simulink model "LQR_Real"  (R2022b)
settings: Solver=VariableStepAuto  StartTime=0.0  StopTime=10  RelTol=1e-3
values from neighbouring files (symbols this model uses):
  beam =     [parameters.mat]
  degs2rpm = 0.166666666667    [parameters.mat]
  Den_tm_wm = [9.422e-10 5.0182e-09 6.49379142857e-06 1.60164591837e-05]    [parameters.mat]
  der =     [parameters.mat]
  drv =     [parameters.mat]
  estimated =     [parameters.mat]
  gbox =     [parameters.mat]
  joint =     [parameters.mat]
  mot =     [parameters.mat]
  Num_tm_wm = [0.0014 0.0034 0.83]    [parameters.mat]
  rads2rpm = 9.54929658551    [parameters.mat]
  rpm2rads = 0.10471975512    [parameters.mat]
  sens =     [parameters.mat]
  Ts = 0.001    [parameters.mat]
undefined symbols (not defined in the file or in its folder): simul, ss_lqr
settings Model: Creator=emanuelevitetta  LastModifiedBy=david

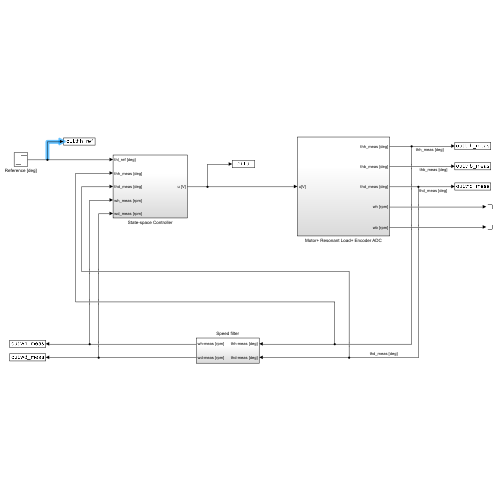
[thumbnail: Simulink's stored preview of the top-level diagram]
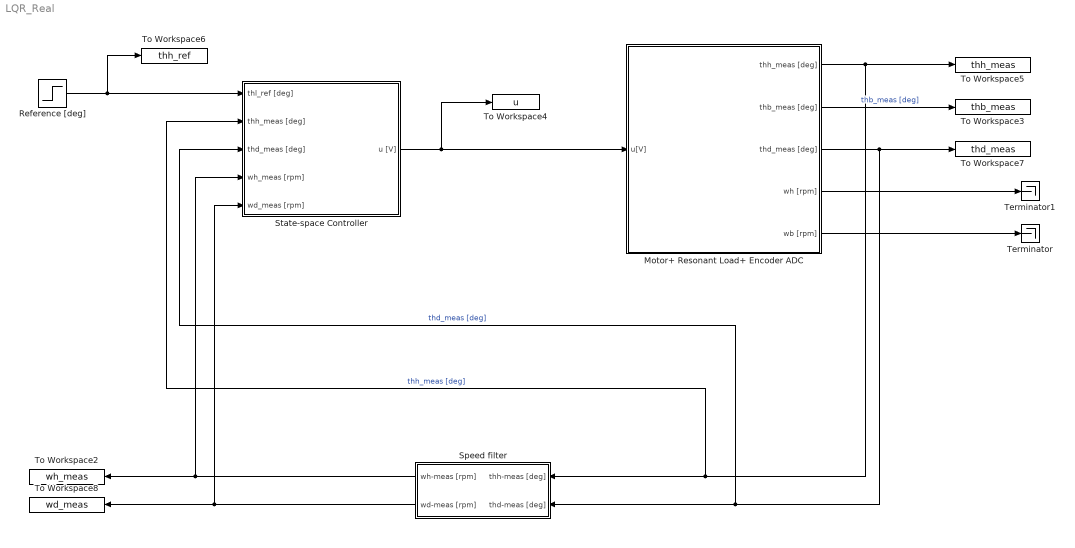
== system LQR_Real ==
  Motor+ Resonant Load+ Encoder ADC : Subsystem
  Reference [deg] : Step  After=simul.stepdeg  SampleTime=Ts
  Speed filter : Subsystem
  State-space Controller : Subsystem
  Terminator : Terminator
  Terminator1 : Terminator
  To Workspace2 : ToWorkspace  VariableName=wh_meas  SaveFormat=Structure With Time  SampleTime=Ts
  To Workspace3 : ToWorkspace  VariableName=thb_meas  SaveFormat=Structure With Time  SampleTime=Ts
  To Workspace4 : ToWorkspace  VariableName=u  SaveFormat=Structure With Time  SampleTime=Ts
  To Workspace5 : ToWorkspace  VariableName=thh_meas  SaveFormat=Structure With Time  SampleTime=Ts
  To Workspace6 : ToWorkspace  VariableName=thh_ref  SaveFormat=Structure With Time  SampleTime=-1
  To Workspace7 : ToWorkspace  VariableName=thd_meas  SaveFormat=Structure With Time  SampleTime=Ts
  To Workspace8 : ToWorkspace  VariableName=wd_meas  SaveFormat=Structure With Time  SampleTime=Ts
  wires:
  Motor+ Resonant Load+ Encoder ADC/1(thh_meas [deg]) -> State-space Controller/2(thh_meas [deg]), Speed filter/1(thh-meas [deg]), To Workspace5/1  "thh_meas [deg]"
  Motor+ Resonant Load+ Encoder ADC/2(thb_meas [deg]) -> To Workspace3/1  "thb_meas [deg]"
  State-space Controller/1(u [V]) -> Motor+ Resonant Load+ Encoder ADC/1(u[V]), To Workspace4/1
  Reference [deg]/1 -> To Workspace6/1, State-space Controller/1(thl_ref [deg])
  Motor+ Resonant Load+ Encoder ADC/5(wb [rpm]) -> Terminator/1
  Motor+ Resonant Load+ Encoder ADC/4(wh [rpm]) -> Terminator1/1
  Motor+ Resonant Load+ Encoder ADC/3(thd_meas [deg]) -> To Workspace7/1, Speed filter/2(thd-meas [deg]), State-space Controller/3(thd_meas [deg])  "thd_meas [deg]"
  Speed filter/2(wd-meas [rpm]) -> State-space Controller/5(wd_meas [rpm]), To Workspace8/1
  Speed filter/1(wh-meas [rpm]) -> State-space Controller/4(wh_meas [rpm]), To Workspace2/1

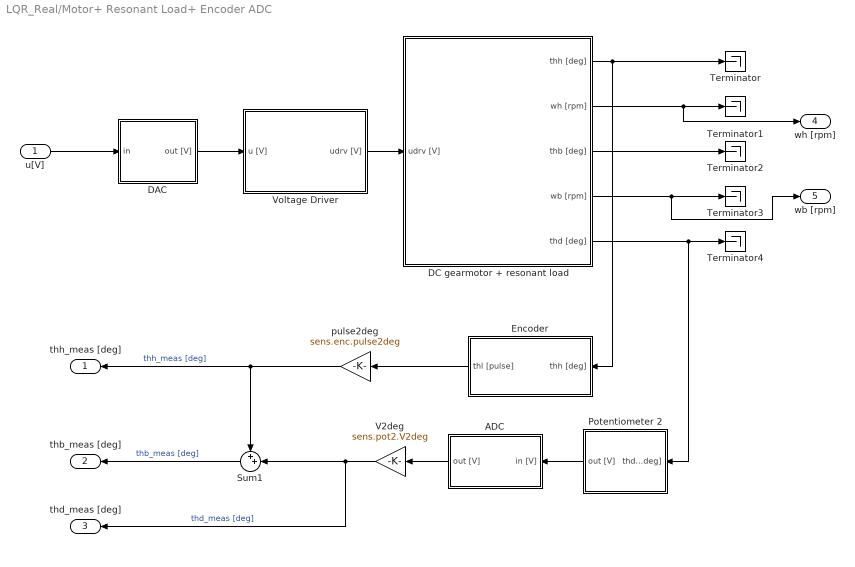
== system LQR_Real/Motor+ Resonant Load+ Encoder ADC ==
  u[V] : Inport
  ADC : Subsystem
  DAC : Subsystem
  DC gearmotor + resonant load : Subsystem
  Encoder : Subsystem
  Potentiometer 2 : Subsystem
  Sum1 : Sum  Inputs=++|
  Terminator{,1..4} (5 alike) : Terminator
  V2deg : Gain  Gain=sens.pot2.V2deg
  Voltage Driver : Subsystem
  pulse2deg : Gain  Gain=sens.enc.pulse2deg
  thh_meas [deg] : Outport
  thb_meas [deg] : Outport  Port=2
  thd_meas [deg] : Outport  Port=3
  wh [rpm] : Outport  Port=4
  wb [rpm] : Outport  Port=5
  wires:
  DC gearmotor + resonant load/2(wh [rpm]) -> wh [rpm]/1, Terminator1/1
  u[V]/1 -> DAC/1(in)
  DC gearmotor + resonant load/1(thh [deg]) -> Terminator/1, Encoder/1(thh [deg])
  DC gearmotor + resonant load/3(thb [deg]) -> Terminator2/1
  DC gearmotor + resonant load/4(wb [rpm]) -> wb [rpm]/1, Terminator3/1
  DC gearmotor + resonant load/5(thd [deg]) -> Terminator4/1, Potentiometer 2/1(thd [deg])
  DAC/1(out [V]) -> Voltage Driver/1(u [V])
  Voltage Driver/1(udrv [V]) -> DC gearmotor + resonant load/1(udrv [V])
  pulse2deg/1 -> thh_meas [deg]/1, Sum1/1  "thh_meas [deg]"
  V2deg/1 -> thd_meas [deg]/1, Sum1/2  "thd_meas [deg]"
  Potentiometer 2/1(out [V]) -> ADC/1(in [V])
  Sum1/1 -> thb_meas [deg]/1  "thb_meas [deg]"
  ADC/1(out [V]) -> V2deg/1
  Encoder/1(thl [pulse]) -> pulse2deg/1

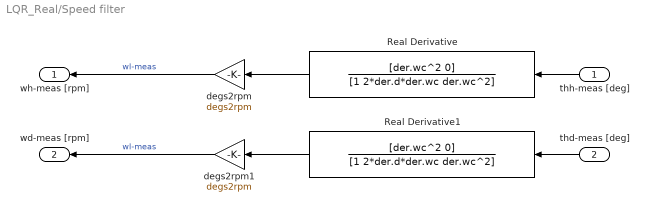
== system LQR_Real/Speed filter ==
  thh-meas [deg] : Inport
  thd-meas [deg] : Inport  Port=2
  Real Derivative : TransferFcn  Numerator=[der.wc^2 0]  Denominator=[1 2*der.d*der.wc der.wc^2]
  Real Derivative1 : TransferFcn  Numerator=[der.wc^2 0]  Denominator=[1 2*der.d*der.wc der.wc^2]
  degs2rpm : Gain  Gain=degs2rpm
  degs2rpm1 : Gain  Gain=degs2rpm
  wh-meas [rpm] : Outport
  wd-meas [rpm] : Outport  Port=2
  wires:
  thh-meas [deg]/1 -> Real Derivative/1
  degs2rpm/1 -> wh-meas [rpm]/1  "wl-meas"
  Real Derivative/1 -> degs2rpm/1
  degs2rpm1/1 -> wd-meas [rpm]/1  "wl-meas"
  Real Derivative1/1 -> degs2rpm1/1
  thd-meas [deg]/1 -> Real Derivative1/1

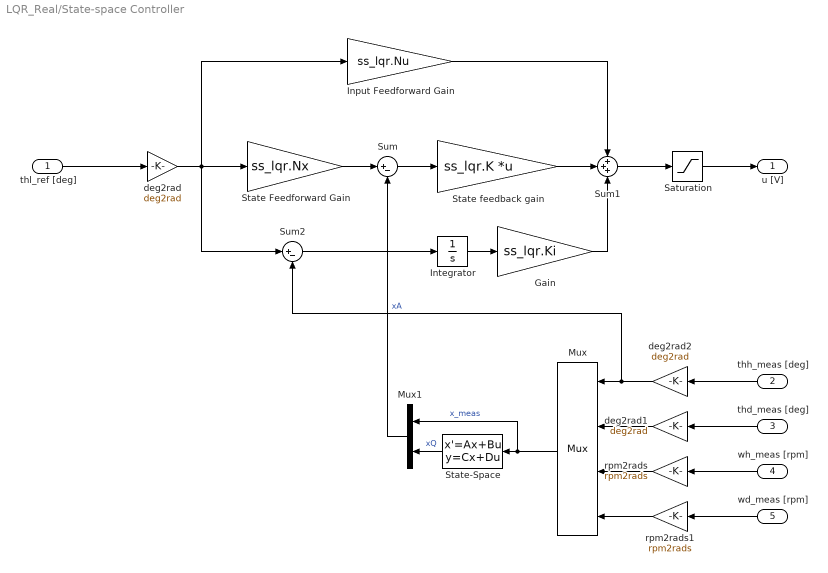
== system LQR_Real/State-space Controller ==
  thl_ref [deg] : Inport
  thh_meas [deg] : Inport  Port=2
  thd_meas [deg] : Inport  Port=3
  wh_meas [rpm] : Inport  Port=4
  wd_meas [rpm] : Inport  Port=5
  Gain : Gain  Gain=ss_lqr.Ki
  Input Feedforward Gain : Gain  Gain=ss_lqr.Nu
  Integrator : Integrator
  Mux : Mux
      settings: DisplayOption=signals
  Mux1 : Mux  Inputs=2
  Saturation : Saturate  UpperLimit=10  LowerLimit=-10
  State Feedforward Gain : Gain  Gain=ss_lqr.Nx
  State feedback gain : Gain  Gain=ss_lqr.K  Multiplication=Matrix(K*u)
  State-Space : StateSpace  A=ss_lqr.AQ  B=ss_lqr.BQ  C=ss_lqr.I  D=ss_lqr.zero  InitialCondition=0
  Sum : Sum  Inputs=|+-
  Sum1 : Sum  Inputs=+++
  Sum2 : Sum  Inputs=|+-
  deg2rad : Gain  Gain=deg2rad
  deg2rad1 : Gain  Gain=deg2rad
  deg2rad2 : Gain  Gain=deg2rad
  rpm2rads : Gain  Gain=rpm2rads
  rpm2rads1 : Gain  Gain=rpm2rads
  u [V] : Outport
  wires:
  thh_meas [deg]/1 -> deg2rad2/1
  wh_meas [rpm]/1 -> rpm2rads/1
  thl_ref [deg]/1 -> deg2rad/1
  deg2rad/1 -> Sum2/1, Input Feedforward Gain/1, State Feedforward Gain/1
  State Feedforward Gain/1 -> Sum/1
  Sum/1 -> State feedback gain/1
  State feedback gain/1 -> Sum1/2
  Sum1/1 -> Saturation/1
  Input Feedforward Gain/1 -> Sum1/1
  deg2rad2/1 -> Sum2/2, Mux/1
  rpm2rads/1 -> Mux/3
  Saturation/1 -> u [V]/1
  thd_meas [deg]/1 -> deg2rad1/1
  deg2rad1/1 -> Mux/2
  wd_meas [rpm]/1 -> rpm2rads1/1
  rpm2rads1/1 -> Mux/4
  Integrator/1 -> Gain/1
  Gain/1 -> Sum1/3
  Sum2/1 -> Integrator/1
  State-Space/1 -> Mux1/2  "xQ"
  Mux/1 -> Mux1/1, State-Space/1  "x_meas"
  Mux1/1 -> Sum/2  "xA"

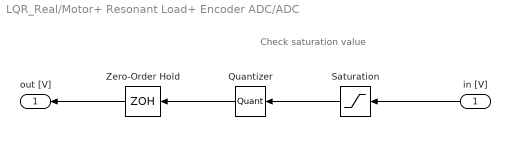
== system LQR_Real/Motor+ Resonant Load+ Encoder ADC/ADC ==
  note: Check saturation value
  in [V] : Inport
  Quantizer : Quantizer  QuantizationInterval=daq.adc.q
  Saturation : Saturate  UpperLimit=10  LowerLimit=-10
  Zero-Order Hold : ZeroOrderHold  SampleTime=Ts
  out [V] : Outport
  wires:
  in [V]/1 -> Saturation/1
  Saturation/1 -> Quantizer/1
  Zero-Order Hold/1 -> out [V]/1
  Quantizer/1 -> Zero-Order Hold/1

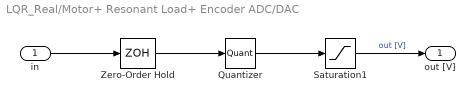
== system LQR_Real/Motor+ Resonant Load+ Encoder ADC/DAC ==
  in : Inport
  Quantizer : Quantizer  QuantizationInterval=daq.dac.q
  Saturation1 : Saturate  UpperLimit=10  LowerLimit=-10
  Zero-Order Hold : ZeroOrderHold  SampleTime=Ts
  out [V] : Outport
  wires:
  Saturation1/1 -> out [V]/1  "out [V]"
  in/1 -> Zero-Order Hold/1
  Zero-Order Hold/1 -> Quantizer/1
  Quantizer/1 -> Saturation1/1

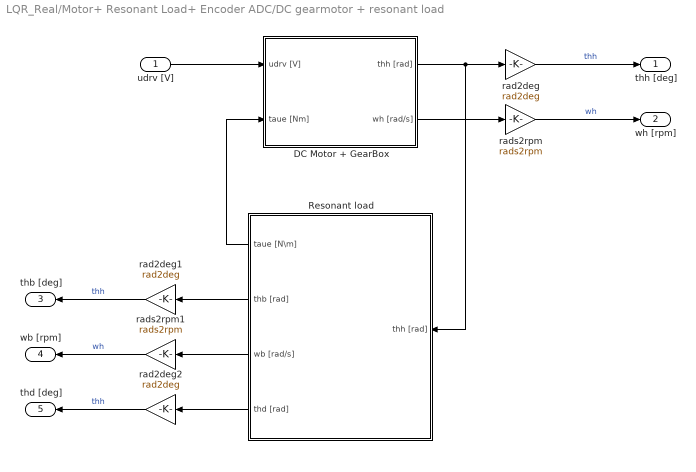
== system LQR_Real/Motor+ Resonant Load+ Encoder ADC/DC gearmotor + resonant load ==
  udrv [V] : Inport
  DC Motor + GearBox : Subsystem
  Resonant load : Subsystem
  rad2deg : Gain  Gain=rad2deg
  rad2deg1 : Gain  Gain=rad2deg
  rad2deg2 : Gain  Gain=rad2deg
  rads2rpm : Gain  Gain=rads2rpm
  rads2rpm1 : Gain  Gain=rads2rpm
  thh [deg] : Outport
  wh [rpm] : Outport  Port=2
  thb [deg] : Outport  Port=3
  wb [rpm] : Outport  Port=4
  thd [deg] : Outport  Port=5
  wires:
  rads2rpm/1 -> wh [rpm]/1  "wh"
  Resonant load/1(taue [N\m]) -> DC Motor + GearBox/2(taue [Nm])
  Resonant load/4(thd [rad]) -> rad2deg2/1
  rads2rpm1/1 -> wb [rpm]/1  "wh"
  DC Motor + GearBox/1(thh [rad]) -> Resonant load/1(thh [rad]), rad2deg/1
  udrv [V]/1 -> DC Motor + GearBox/1(udrv [V])
  rad2deg1/1 -> thb [deg]/1  "thh"
  Resonant load/3(wb [rad/s]) -> rads2rpm1/1
  DC Motor + GearBox/2(wh [rad/s]) -> rads2rpm/1
  rad2deg/1 -> thh [deg]/1  "thh"
  Resonant load/2(thb [rad]) -> rad2deg1/1
  rad2deg2/1 -> thd [deg]/1  "thh"

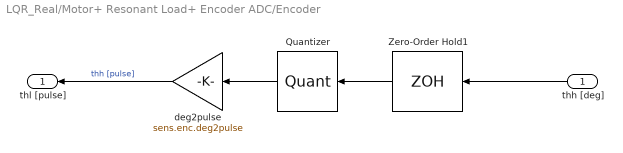
== system LQR_Real/Motor+ Resonant Load+ Encoder ADC/Encoder ==
  thh [deg] : Inport
  Quantizer : Quantizer  QuantizationInterval=sens.enc.pulse2deg
  Zero-Order Hold1 : ZeroOrderHold  SampleTime=Ts
  deg2pulse : Gain  Gain=sens.enc.deg2pulse
  thl [pulse] : Outport
  wires:
  thh [deg]/1 -> Zero-Order Hold1/1
  Zero-Order Hold1/1 -> Quantizer/1
  deg2pulse/1 -> thl [pulse]/1  "thh [pulse]"
  Quantizer/1 -> deg2pulse/1

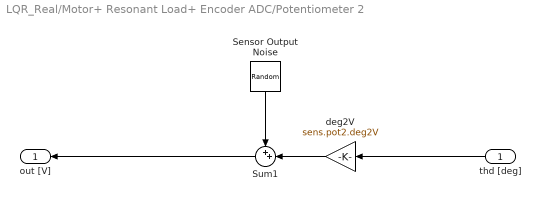
== system LQR_Real/Motor+ Resonant Load+ Encoder ADC/Potentiometer 2 ==
  thd [deg] : Inport
  Sensor Output Noise : RandomNumber  Variance=sens.pot2.var  SampleTime=Ts
  Sum1 : Sum  Inputs=++|
  deg2V : Gain  Gain=sens.pot2.deg2V
  out [V] : Outport
  wires:
  Sum1/1 -> out [V]/1
  thd [deg]/1 -> deg2V/1
  Sensor Output Noise/1 -> Sum1/1
  deg2V/1 -> Sum1/2

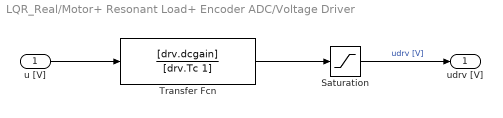
== system LQR_Real/Motor+ Resonant Load+ Encoder ADC/Voltage Driver ==
  u [V] : Inport
  Saturation : Saturate  UpperLimit=12  LowerLimit=-12
  Transfer Fcn : TransferFcn  Numerator=[drv.dcgain]  Denominator=[drv.Tc 1]
  udrv [V] : Outport
  wires:
  Saturation/1 -> udrv [V]/1  "udrv [V]"
  u [V]/1 -> Transfer Fcn/1
  Transfer Fcn/1 -> Saturation/1

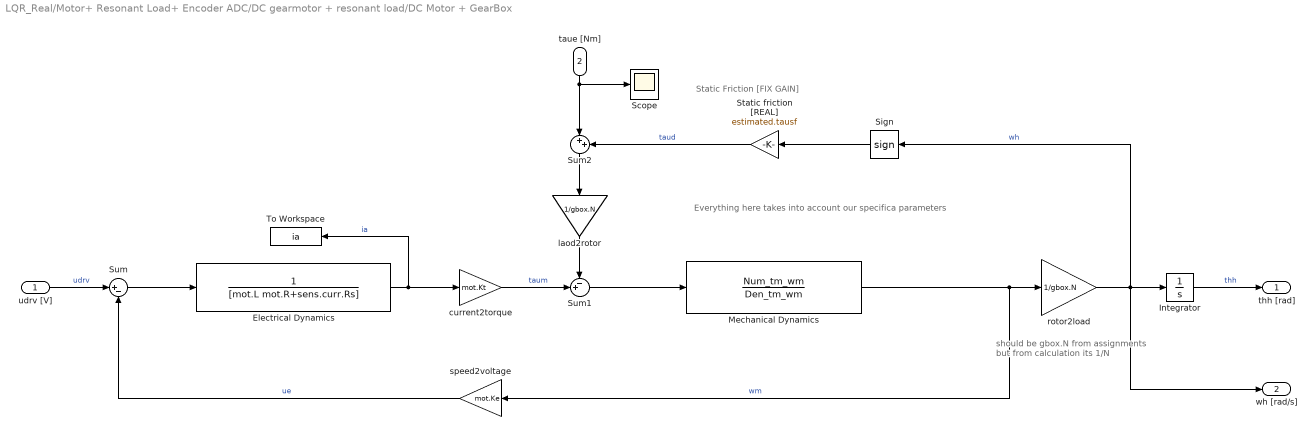
== system LQR_Real/Motor+ Resonant Load+ Encoder ADC/DC gearmotor + resonant load/DC Motor + GearBox ==
  note: Everything here takes into account our specifica parameters
  note: Static Friction [FIX GAIN]
  note: should be gbox.N from assignments
      | but from calculation its 1/N
  udrv [V] : Inport
  taue [Nm] : Inport  Port=2
  Electrical Dynamics : TransferFcn  Denominator=[mot.L mot.R+sens.curr.Rs]
  Integrator : Integrator  IgnoreLimit=on
  Mechanical Dynamics : TransferFcn  Numerator=Num_tm_wm  Denominator=Den_tm_wm
  Scope : Scope
  Sign : Signum  ZeroCross=off
  Static friction [REAL] : Gain  Gain=estimated.tausf
  Sum : Sum  Inputs=|+-
  Sum1 : Sum  Inputs=-+|
  Sum2 : Sum  Inputs=|++
  To Workspace : ToWorkspace  VariableName=ia  SaveFormat=Structure With Time  SampleTime=-1
  current2torque : Gain  Gain=mot.Kt
  laod2rotor : Gain  Gain=1/gbox.N
  rotor2load : Gain  Gain=1/gbox.N
  speed2voltage : Gain  Gain=mot.Ke
  thh [rad] : Outport
  wh [rad/s] : Outport  Port=2
  wires:
  Sign/1 -> Static friction [REAL]/1
  Electrical Dynamics/1 -> current2torque/1, To Workspace/1  "ia"
  Sum1/1 -> Mechanical Dynamics/1
  rotor2load/1 -> wh [rad/s]/1, Sign/1, Integrator/1  "wh"
  laod2rotor/1 -> Sum1/1
  udrv [V]/1 -> Sum/1  "udrv"
  current2torque/1 -> Sum1/2  "taum"
  speed2voltage/1 -> Sum/2  "ue"
  Sum/1 -> Electrical Dynamics/1
  Sum2/1 -> laod2rotor/1
  Static friction [REAL]/1 -> Sum2/2  "taud"
  taue [Nm]/1 -> Sum2/1, Scope/1
  Integrator/1 -> thh [rad]/1  "thh"
  Mechanical Dynamics/1 -> speed2voltage/1, rotor2load/1  "wm"

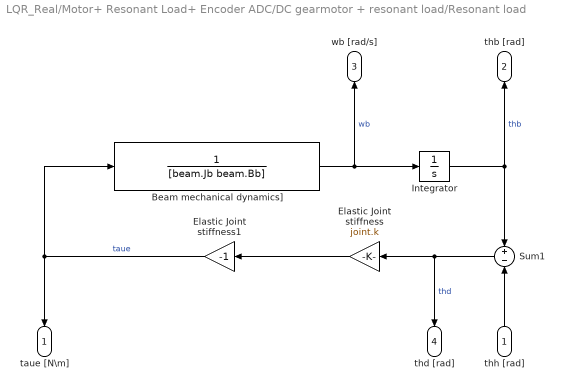
== system LQR_Real/Motor+ Resonant Load+ Encoder ADC/DC gearmotor + resonant load/Resonant load ==
  thh [rad] : Inport
  Beam mechanical dynamics] : TransferFcn  Denominator=[beam.Jb beam.Bb]
  Elastic Joint stiffness : Gain  Gain=joint.k
  Elastic Joint stiffness1 : Gain  Gain=-1
  Integrator : Integrator
  Sum1 : Sum  Inputs=+-
  taue [N\m] : Outport
  thb [rad] : Outport  Port=2
  wb [rad/s] : Outport  Port=3
  thd [rad] : Outport  Port=4
  wires:
  thh [rad]/1 -> Sum1/2
  Beam mechanical dynamics]/1 -> wb [rad/s]/1, Integrator/1  "wb"
  Sum1/1 -> thd [rad]/1, Elastic Joint stiffness/1  "thd"
  Elastic Joint stiffness/1 -> Elastic Joint stiffness1/1
  Elastic Joint stiffness1/1 -> Beam mechanical dynamics]/1, taue [N\m]/1  "taue"
  Integrator/1 -> thb [rad]/1, Sum1/1  "thb"
